simulink model "receive_a664_r2020b"  (R2020b)
settings: Solver=VariableStepAuto  StartTime=0.0  StopTime=10.0  RelTol=1e-3
model workspace (MAT data in the model file):
  ED247Configuration.ECICFile = 'C:\Files\SANDBOX\git\ED247\ed247_for_simulink\tests\_files\ecic\ecic_func_exchange_a664_uc_tester.xml'
  ED247Configuration.ICDFiles = {'C:\Files\SANDBOX\git\ED247\ed247_for_simulink\tests\_files\ecic\icd_func_exchange_a664_uc_tester.xml'}
  ED247Configuration.Configuration.name = 'T11MX_15430_TEST_STEP_O'
  ED247Configuration.Configuration.direction = 'IN'
  ED247Configuration.Configuration.type = 'uint8'
  ED247Configuration.Configuration.dimensions = 1
  ED247Configuration.Configuration.width = 4
  ED247Configuration.Configuration.size = 4
  ED247Configuration.Configuration.sample_time = 1
  ED247Configuration.Configuration.validity_duration = 1
  ED247Configuration.Configuration.signal_type = 'A664'
  ED247Configuration.Configuration.sample_size = 4
libraries: lib_ed247 x2
settings Model: OrderedModelArguments=off  Creator=odufour  LastModifiedBy=odufour
settings DebuggingCC: InheritedTsInSrcMsg=none

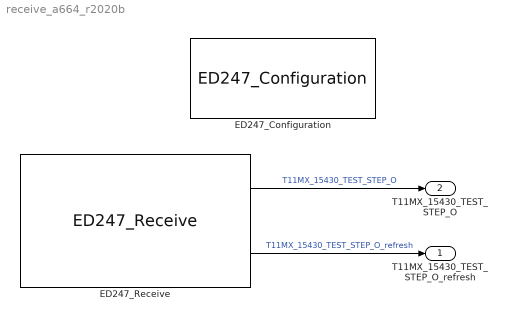
== system receive_a664_r2020b ==
  ED247_Configuration : lib_ed247/ED247_Configuration  configurationFilename='ecic_func_exchange_a664_uc_tester.xml'  enableLog=off  logFilename=''
      settings: SourceProductName=Airbus ED247
  ED247_Receive : lib_ed247/ED247_Receive  enable_refresh=on  refresh_factor=1  sample_time=-1  show_port_labels=on
      settings: SourceProductName=Airbus ED247
  T11MX_15430_TEST_STEP_O_refresh : Outport
  T11MX_15430_TEST_STEP_O : Outport  Port=2  OutDataTypeStr=uint8  PortDimensions=4  SampleTime=0.1
  wires:
  ED247_Receive/1 -> T11MX_15430_TEST_STEP_O/1  "T11MX_15430_TEST_STEP_O"
  ED247_Receive/2 -> T11MX_15430_TEST_STEP_O_refresh/1  "T11MX_15430_TEST_STEP_O_refresh"
